simulink model "Auxiliary_Models"  (R2020b)
settings: Solver=VariableStepAuto  StartTime=0.0  StopTime=10.0  RelTol=1e-3
undefined symbols (not defined in the file or in its folder): Actuators, ampl_p_cmd, ARI, beta_cmd, Ki, Klp, Klz, Kp, Kr, omega_lp, omega_p_cmd, omega_wo, TestSequence, TrimPoint, TurnCompensation
libraries: simulink x29
settings Model: Creator=NicolasS  LastModifiedBy=NicolasS

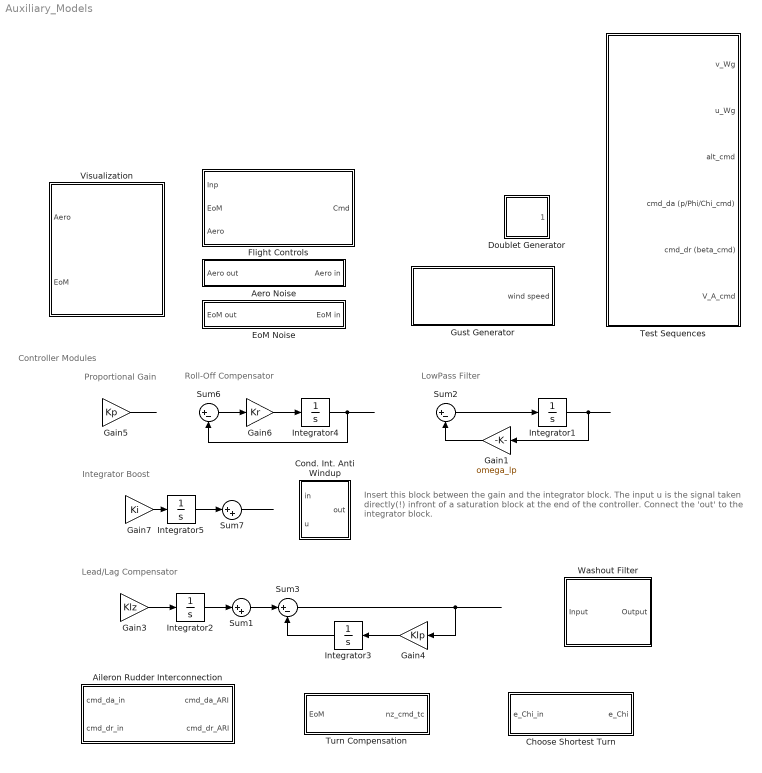
== system Auxiliary_Models ==
  note: Insert this block between the gain and the integrator block.
      | The input u is the signal taken directly(!) infront of a saturation block at the end of the controller. Connect the 'out' to the integrator block.
  note: Controller Modules
  note: Integrator Boost
  note: Roll-Off Compensator
  note: Proportional
      | Gain
  note: Lead/Lag Compensator
  note: LowPass Filter
  Aero Noise : Subsystem
  Aileron Rudder Interconnection : Subsystem
  Choose Shortest Turn : MATLAB Function  TreatAsAtomicUnit=on
  Cond. Int. Anti Windup : Subsystem  mask(Integrator Anti-Windup){max_u=inf, min_u=-inf, negative_sign=off}
      mask prompts: max_u "Maximum control signal"; min_u "Minimum control signal"; negative_sign "Negative amplification in control law"
      mask help:
      | This block provides integration using the "conditional integration" anti-windup compensation.
      | It compares the sign of the error and the sign of the control signal and stops integration in case the error drives saturation.
      mask Help:
      | This block provides integration using the "conditional integration" anti-windup compensation. It stops or continues integration depending on the sign of the integrator input (control error) and the commanded control signal. Only if the input would further increase the already saturated integrator output, integration is stopped. This method is different from "integrator clamping" and and "integrator back calculation" and usually provides better recovery properties.
      | 
      | In a standard control architecture the inputs are as follows:
      | INPUT is the error signal r-y
      | RESET is a reset signal. The integrator state is reseted on either rising or falling edges
      | X0 is the initial condition for the integrator
      | U is the commanded control signal
      | 
      | For the anti-windup to work as intended, a saturation block must be placed on the ouput of the control command being fed to the associated actuator, which should include all control signal contributions (e.g. from proportional feedback and inner loops). U is the signal before this saturation.
      | 
      | The default logic assumes a plant with positive steady-state gain to be controlled. This translates to the following logic:
      | For commanded control signal u, saturation limits Umax and Umin, and error e,
      | If u is in bounds, do nothing
      | If u >= Umax AND e > 0, stop integrating
      | If u >= Umax AND e < 0, continue integrating
      | If u <= Umin AND e > 0, continue integrating
      | If u <= Umin AND e < 0, stop integrating
      | 
      | If a plant with negative steady-state gain is to be controlled (e.g. pitch), the windup logic may changed using the NEGATIVE SIGN option. (Note: If unsure check if the controller gains are negative. If yes, check the NEGATIVE SIGN option)
      | This then translates to the logic:
      | If u is in bounds, do nothing
      | If u >= Umax AND e < 0, stop integrating
      | If u >= Umax AND e > 0, continue integrating
      | If u <= Umin AND e < 0, continue integrating
      | If u <= Umin AND e > 0, stop integrating
  Doublet Generator : Subsystem  mask(DoubletGenerator){timeon=0, pulsewidth=1, amplitude=1}
      mask prompts: timeon "Time Start"; pulsewidth "Pulse Duration"
      mask help:
      | Doublet Generator.
      | Ouputs doublet of specificed amplitude and duration.
      |
      | If start/duration/amplitude parameters are vectors, then output is multichannel.
      mask Display: plot([.1 .3 .3001 .4 .4001 .5  .5001 .7],[0 0 1 1 -1 -1 0 0])
  EoM Noise : Subsystem
  Flight Controls : Subsystem
  Gain1 : Gain  Gain=omega_lp
  Gain3 : Gain  Gain=Klz
  Gain4 : Gain  Gain=Klp
  Gain5 : Gain  Gain=Kp
  Gain6 : Gain  Gain=Kr
  Gain7 : Gain  Gain=Ki
  Gust Generator : Subsystem  mask{gust_start=0, gust_duration=0, gust_amplitude=0}
      mask prompts: gust_start "start time of the gust in sec"; gust_duration "gust duration in sec"; gust_amplitude "maximum gust speed in m/s"
      mask DialogControl ParameterGroupVar Prompt: gust characteristics
  Integrator{1..5} (5 alike) : Integrator  UpperSaturationLimit=max(Actuators.Limits.u_max_He)  LowerSaturationLimit=min(Actuators.Limits.u_max_He)  ContinuousStateAttributes='K'
  Sum1 : Sum  Inputs=|++
  Sum2 : Sum  Inputs=|+-
  Sum3 : Sum  Inputs=|+-
  Sum6 : Sum  Inputs=|+-
  Sum7 : Sum  Inputs=|++
  Test Sequences : Subsystem  InitFcn=|  StopFcn="clear beta_cmd  ampl_p_cmd omega_p_cmd tstart_p_cmd tstart_p_cmd TurnCompensation"
      | if not(exist('TestSequence','var'))
      | TestSequence = 7;
      | end
      | 
      | if not(exist('beta_cmd','var'))
      | beta_cmd = 0;
      | end
      | 
      | if not(exist('ampl_p_cmd','var'))
      | ampl_p_cmd = 0;
      | end
      | 
      | if not(exist('omega_p_cmd','var'))
      | omega_p_cmd = 0;
      | end
      | 
      | if not(exist('tstart_p_cmd','var'))
      | tstart_p_cmd = 0;
      | end
      | 
      | if not(exist('TurnCompensation','var'))
      |  if TestSequence == 4
      |     TurnCompensation = 0;
      |  else
      |     TurnCompensation = 1;
      |  end
      | end
  Turn Compensation : Subsystem
  Visualization : Subsystem
  Washout Filter : Subsystem  mask{wb=omega_wo}
      mask prompts: wb "Filter Bandwidth"
      mask Display:
      | plot([0.35 0.5 0.65 ],[0.4 0.6 0.6 ]);
      | text(0.5,0.3,[num2str(wb) ' rad/s'],'horizontalAlignment', 'center');
      | text(0.67,0.6,['1'],'horizontalAlignment', 'left');
  wires:
  Sum7/1 -> ?
  Gain7/1 -> Integrator5/1
  Sum6/1 -> Gain6/1
  Integrator5/1 -> Sum7/1
  Gain6/1 -> Integrator4/1
  ? -> Gain5/1
  ? -> Gain7/1, Sum7/2
  Gain5/1 -> ?
  ? -> Sum6/1
  Integrator4/1 -> Sum6/2
  ? -> Sum1/2, Gain3/1
  Integrator2/1 -> Sum1/1
  Sum1/1 -> Sum3/1
  Gain4/1 -> Integrator3/1
  Integrator3/1 -> Sum3/2
  Sum3/1 -> Gain4/1
  Gain3/1 -> Integrator2/1
  Gain1/1 -> Sum2/2
  Sum2/1 -> Integrator1/1
  Integrator1/1 -> Gain1/1
  ? -> Sum2/1

== system Auxiliary_Models/Aero Noise ==
  Aero in : Inport  OutDataTypeStr=Bus: Aero
  Band-Limited White Noise1 : simulink/Sources/Band-Limited White Noise  Cov=1E-7  Ts=0.01  seed=5749
  Band-Limited White Noise8 : simulink/Sources/Band-Limited White Noise  Cov=1E-7  Ts=0.01  seed=3324
  Band-Limited White Noise9 : simulink/Sources/Band-Limited White Noise  Cov=1E-3  Ts=0.05  seed=8153
  Bus Creator2 : BusCreator  Inputs=7  OutDataTypeStr=Bus: Aero
  Bus Creator3 : BusCreator  Inputs=7  OutDataTypeStr=Bus: AirData
  Bus Selector : BusSelector  OutputSignals=AirData.u_Af,AirData.v_Af,AirData.w_Af,AirData.V_A,AirData.p_dyn,AirData.alpha,AirData.beta,X_A,Y_A,Z_A,L_A,M_A,N_A
  Sum1 : Sum  Inputs=++|
  Sum2 : Sum  Inputs=++|
  Sum3 : Sum  Inputs=++|
  Aero out : Outport  OutDataTypeStr=Bus: Aero
  wires:
  Aero in/1 -> Bus Selector/1
  Bus Creator3/1 -> Bus Creator2/1  "AirData"
  Bus Selector/7 -> Sum2/2  "<beta>"
  Bus Selector/8 -> Bus Creator2/2  "<X_A>"
  Bus Creator2/1 -> Aero out/1  "Aero"
  Bus Selector/1 -> Bus Creator3/1  "<u_Af>"
  Bus Selector/3 -> Bus Creator3/3  "<w_Af>"
  Bus Selector/4 -> Sum3/2  "<V_A>"
  Bus Selector/6 -> Sum1/2  "<alpha>"
  Band-Limited White Noise8/1 -> Sum1/1
  Sum1/1 -> Bus Creator3/6  "alpha"
  Bus Selector/5 -> Bus Creator3/5  "<p_dyn>"
  Band-Limited White Noise9/1 -> Sum3/1
  Sum3/1 -> Bus Creator3/4  "V_A"
  Bus Selector/2 -> Bus Creator3/2  "<v_Af>"
  Bus Selector/9 -> Bus Creator2/3  "<Y_A>"
  Bus Selector/10 -> Bus Creator2/4  "<Z_A>"
  Bus Selector/11 -> Bus Creator2/5  "<L_A>"
  Bus Selector/12 -> Bus Creator2/6  "<M_A>"
  Bus Selector/13 -> Bus Creator2/7  "<N_A>"
  Band-Limited White Noise1/1 -> Sum2/1
  Sum2/1 -> Bus Creator3/7  "beta"

== system Auxiliary_Models/Aileron Rudder Interconnection ==
  cmd_da_in : Inport
  cmd_dr_in : Inport  Port=2
  ARI : Constant  Value=ARI
  Demux : Demux  Outputs=2
  Mux : Mux  Inputs=2
  Product : Product  Multiplication=Matrix(*)
  cmd_da_ARI : Outport
  cmd_dr_ARI : Outport  Port=2
  wires:
  cmd_da_in/1 -> Mux/1
  ARI/1 -> Product/1
  Demux/1 -> cmd_da_ARI/1
  Demux/2 -> cmd_dr_ARI/1
  Product/1 -> Demux/1
  cmd_dr_in/1 -> Mux/2
  Mux/1 -> Product/2

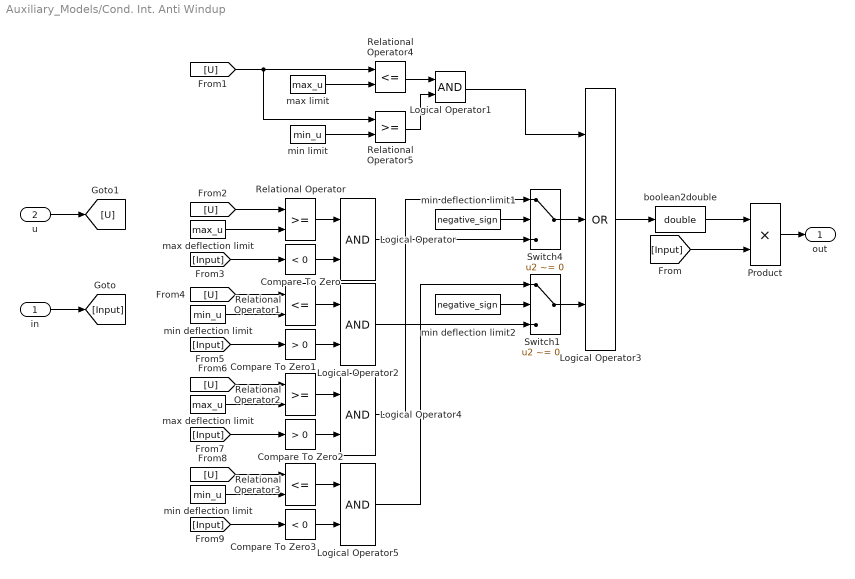
== system Auxiliary_Models/Cond. Int. Anti Windup ==
  in : Inport
  u : Inport  Port=2
  Compare To Zero : simulink/Logic and Bit Operations/Compare To Zero  relop=<  OutDataTypeStr=uint8
  Compare To Zero1 : simulink/Logic and Bit Operations/Compare To Zero  relop=>  OutDataTypeStr=uint8
  Compare To Zero2 : simulink/Logic and Bit Operations/Compare To Zero  relop=>  OutDataTypeStr=uint8
  Compare To Zero3 : simulink/Logic and Bit Operations/Compare To Zero  relop=<  OutDataTypeStr=uint8
  Logical Operator{,1..2,4..5} (5 alike) : Logic  AllPortsSameDT=off  OutDataTypeStr=boolean
  Logical Operator3 : Logic  Operator=OR  Inputs=3  AllPortsSameDT=off  OutDataTypeStr=boolean
  Product : Product
  Relational Operator : RelationalOperator  OutDataTypeStr=boolean  RndMeth=Nearest
  Relational Operator1 : RelationalOperator  Operator=<=  OutDataTypeStr=boolean  RndMeth=Nearest
  Relational Operator2 : RelationalOperator  OutDataTypeStr=boolean  RndMeth=Nearest
  Relational Operator3 : RelationalOperator  Operator=<=  OutDataTypeStr=boolean  RndMeth=Nearest
  Relational Operator4 : RelationalOperator  Operator=<=  OutDataTypeStr=boolean  RndMeth=Nearest
  Relational Operator5 : RelationalOperator  OutDataTypeStr=boolean  RndMeth=Nearest
  Switch1 : Switch  Criteria=u2 ~= 0
  Switch4 : Switch  Criteria=u2 ~= 0
  boolean2double : DataTypeConversion  OutDataTypeStr=double
  max deflection limit : Constant  Value=max_u  SampleTime=-1
  "max deflection limit " : Constant  Value=max_u  SampleTime=-1
  max limit : Constant  Value=max_u  SampleTime=-1
  min deflection limit : Constant  Value=min_u  SampleTime=-1
  "min deflection limit " : Constant  Value=min_u  SampleTime=-1
  min deflection limit1 : Constant  Value=negative_sign  SampleTime=-1
  min deflection limit2 : Constant  Value=negative_sign  SampleTime=-1
  min limit : Constant  Value=min_u  SampleTime=-1
  out : Outport
  wires:
  Product/1 -> out/1
  Logical Operator3/1 -> boolean2double/1
  boolean2double/1 -> Product/1
  [Input] -> Product/2
  [Input] -> Compare To Zero3/1
  [U] -> Relational Operator3/1
  [Input] -> Compare To Zero2/1
  [U] -> Relational Operator2/1
  [Input] -> Compare To Zero1/1
  [U] -> Relational Operator1/1
  [Input] -> Compare To Zero/1
  [U] -> Relational Operator/1
  [U] -> Relational Operator4/1, Relational Operator5/1
  u/1 -> [U]
  in/1 -> [Input]
  min limit/1 -> Relational Operator5/2
  Relational Operator5/1 -> Logical Operator1/2
  Relational Operator4/1 -> Logical Operator1/1
  max limit/1 -> Relational Operator4/2
  Logical Operator5/1 -> Switch1/1
  Logical Operator4/1 -> Switch4/1
  Logical Operator2/1 -> Switch1/3
  Logical Operator/1 -> Switch4/3
  min deflection limit1/1 -> Switch4/2
  Switch1/1 -> Logical Operator3/3
  min deflection limit2/1 -> Switch1/2
  max deflection limit/1 -> Relational Operator/2
  Compare To Zero/1 -> Logical Operator/2
  Relational Operator/1 -> Logical Operator/1
  Compare To Zero1/1 -> Logical Operator2/2
  Relational Operator1/1 -> Logical Operator2/1
  min deflection limit/1 -> Relational Operator1/2
  Switch4/1 -> Logical Operator3/2
  Logical Operator1/1 -> Logical Operator3/1
  Compare To Zero2/1 -> Logical Operator4/2
  Relational Operator2/1 -> Logical Operator4/1
  Compare To Zero3/1 -> Logical Operator5/2
  Relational Operator3/1 -> Logical Operator5/1
  "min deflection limit "/1 -> Relational Operator3/2
  "max deflection limit "/1 -> Relational Operator2/2

== system Auxiliary_Models/Doublet Generator ==
  Add : Sum  Inputs=+++
  DownStep : Step  Time=timeon+pulsewidth  After=-2  SampleTime=0
  Gain : Gain  Gain=amplitude
  UnStep : Step  Time=timeon+2*pulsewidth  SampleTime=0
  UpStep : Step  Time=timeon  SampleTime=0
  Doublet : Outport
  wires:
  UpStep/1 -> Add/1
  DownStep/1 -> Add/2
  UnStep/1 -> Add/3
  Add/1 -> Gain/1
  Gain/1 -> Doublet/1

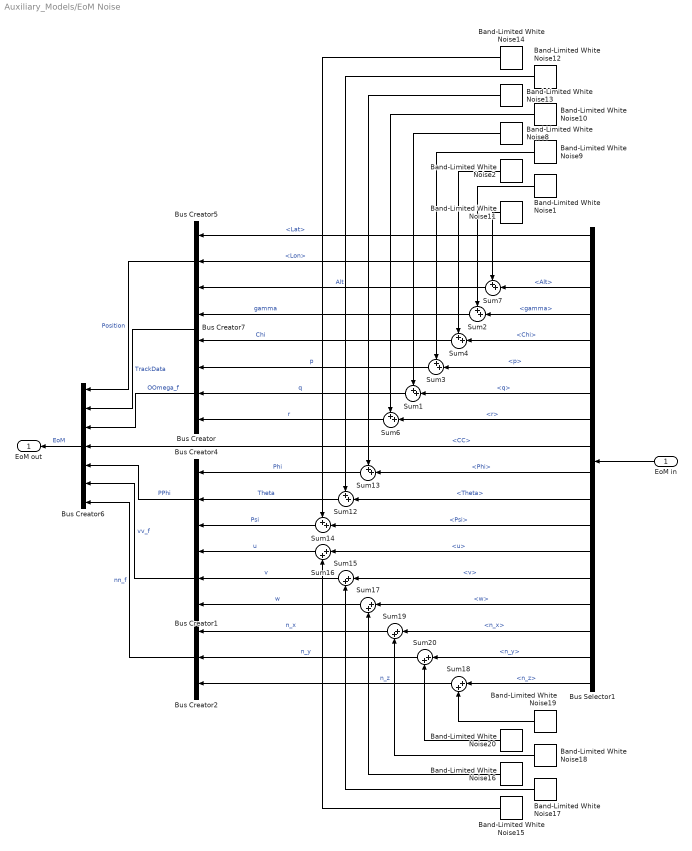
== system Auxiliary_Models/EoM Noise ==
  EoM in : Inport  OutDataTypeStr=Bus: EoM
  Band-Limited White Noise1 : simulink/Sources/Band-Limited White Noise  Cov=1E-7  Ts=0.01  seed=1102
  Band-Limited White Noise10 : simulink/Sources/Band-Limited White Noise  Cov=1E-6  Ts=0.01  seed=66897
  Band-Limited White Noise11 : simulink/Sources/Band-Limited White Noise  Cov=1E-4  Ts=0.1  seed=6874
  Band-Limited White Noise12 : simulink/Sources/Band-Limited White Noise  Cov=5E-7  Ts=0.01  seed=45875
  Band-Limited White Noise13 : simulink/Sources/Band-Limited White Noise  Cov=5E-7  Ts=0.01  seed=74148
  Band-Limited White Noise14 : simulink/Sources/Band-Limited White Noise  Cov=5E-7  Ts=0.01  seed=3514
  Band-Limited White Noise15 : simulink/Sources/Band-Limited White Noise  Cov=5E-5  Ts=0.1  seed=54769
  Band-Limited White Noise16 : simulink/Sources/Band-Limited White Noise  Cov=1E-4  Ts=0.01  seed=6932
  Band-Limited White Noise17 : simulink/Sources/Band-Limited White Noise  Cov=1E-4  Ts=0.01  seed=4485
  Band-Limited White Noise18 : simulink/Sources/Band-Limited White Noise  Cov=1E-5  Ts=0.01  seed=11452
  Band-Limited White Noise19 : simulink/Sources/Band-Limited White Noise  Cov=1E-5  Ts=0.01  seed=3324
  Band-Limited White Noise2 : simulink/Sources/Band-Limited White Noise  Cov=1E-7  Ts=0.1  seed=2201
  Band-Limited White Noise20 : simulink/Sources/Band-Limited White Noise  Cov=1E-5  Ts=0.01  seed=58967
  Band-Limited White Noise8 : simulink/Sources/Band-Limited White Noise  Cov=1E-6  Ts=0.01  seed=[23341]
  Band-Limited White Noise9 : simulink/Sources/Band-Limited White Noise  Cov=1E-6  Ts=0.01  seed=1147
  Bus Creator : BusCreator  Inputs=3  OutDataTypeStr=Bus: OOmega_f
  Bus Creator1 : BusCreator  Inputs=3  OutDataTypeStr=Bus: vv_f
  Bus Creator2 : BusCreator  Inputs=3  OutDataTypeStr=Bus: nn_f
  Bus Creator4 : BusCreator  Inputs=3  OutDataTypeStr=Bus: PPhi
  Bus Creator5 : BusCreator  Inputs=3  OutDataTypeStr=Bus: Position
  Bus Creator6 : BusCreator  Inputs=7  OutDataTypeStr=Bus: EoM
  Bus Creator7 : BusCreator  Inputs=2  OutDataTypeStr=Bus: TrackData
  Bus Selector1 : BusSelector  OutputSignals=Position.Lat,Position.Lon,Position.Alt,TrackData.gamma,TrackData.Chi,OOmega_f.p,OOmega_f.q,OOmega_f.r,CC,PPhi.Phi,PPhi.Theta,PPhi.Psi,vv_f.u,vv_f.v,vv_f.w,nn_f.n_x,nn_f.n_y,nn_f.n_z
  Sum{1..4,6..7,12..14} (9 alike) : Sum  Inputs=++|
  Sum{15..20} (6 alike) : Sum  Inputs=|++
  EoM out : Outport  OutDataTypeStr=Bus: EoM
  wires:
  EoM in/1 -> Bus Selector1/1
  Bus Selector1/6 -> Sum3/2  "<p>"
  Bus Selector1/7 -> Sum1/2  "<q>"
  Band-Limited White Noise9/1 -> Sum3/1
  Bus Selector1/8 -> Sum6/2  "<r>"
  Band-Limited White Noise10/1 -> Sum6/1
  Band-Limited White Noise11/1 -> Sum7/1
  Bus Selector1/3 -> Sum7/2  "<Alt>"
  Band-Limited White Noise12/1 -> Sum12/1
  Bus Selector1/10 -> Sum13/2  "<Phi>"
  Bus Selector1/11 -> Sum12/2  "<Theta>"
  Bus Selector1/12 -> Sum14/2  "<Psi>"
  Band-Limited White Noise13/1 -> Sum13/1
  Band-Limited White Noise14/1 -> Sum14/1
  Bus Selector1/16 -> Sum19/1  "<n_x>"
  Bus Selector1/17 -> Sum20/1  "<n_y>"
  Bus Selector1/18 -> Sum18/1  "<n_z>"
  Bus Selector1/15 -> Sum17/1  "<w>"
  Bus Selector1/13 -> Sum16/1  "<u>"
  Band-Limited White Noise16/1 -> Sum17/2
  Band-Limited White Noise15/1 -> Sum16/2
  Bus Selector1/14 -> Sum15/1  "<v>"
  Band-Limited White Noise17/1 -> Sum15/2
  Band-Limited White Noise19/1 -> Sum18/2
  Band-Limited White Noise18/1 -> Sum19/2
  Band-Limited White Noise20/1 -> Sum20/2
  Bus Selector1/1 -> Bus Creator5/1  "<Lat>"
  Bus Selector1/2 -> Bus Creator5/2  "<Lon>"
  Sum19/1 -> Bus Creator2/1  "n_x"
  Sum20/1 -> Bus Creator2/2  "n_y"
  Sum18/1 -> Bus Creator2/3  "n_z"
  Sum15/1 -> Bus Creator1/2  "v"
  Sum16/1 -> Bus Creator1/1  "u"
  Sum17/1 -> Bus Creator1/3  "w"
  Sum7/1 -> Bus Creator5/3  "Alt"
  Sum6/1 -> Bus Creator/3  "r"
  Sum1/1 -> Bus Creator/2  "q"
  Sum3/1 -> Bus Creator/1  "p"
  Sum13/1 -> Bus Creator4/1  "Phi"
  Bus Selector1/9 -> Bus Creator6/4  "<CC>"
  Sum12/1 -> Bus Creator4/2  "Theta"
  Sum14/1 -> Bus Creator4/3  "Psi"
  Bus Creator5/1 -> Bus Creator6/1  "Position"
  Bus Creator/1 -> Bus Creator6/3  "OOmega_f"
  Bus Creator4/1 -> Bus Creator6/5  "PPhi"
  Bus Creator1/1 -> Bus Creator6/6  "vv_f"
  Bus Creator2/1 -> Bus Creator6/7  "nn_f"
  Bus Creator6/1 -> EoM out/1  "EoM"
  Band-Limited White Noise8/1 -> Sum1/1
  Bus Creator7/1 -> Bus Creator6/2  "TrackData"
  Band-Limited White Noise1/1 -> Sum2/1
  Bus Selector1/5 -> Sum4/2  "<Chi>"
  Band-Limited White Noise2/1 -> Sum4/1
  Bus Selector1/4 -> Sum2/2  "<gamma>"
  Sum2/1 -> Bus Creator7/1  "gamma"
  Sum4/1 -> Bus Creator7/2  "Chi"

== system Auxiliary_Models/Flight Controls ==
  Inp : Inport
  EoM : Inport  Port=2  OutDataTypeStr=Bus: EoM
  Aero : Inport  Port=3  OutDataTypeStr=Bus: Aero
  Bus Creator1 : BusCreator  Inputs=4  OutDataTypeStr=Bus: Cmd
  Lateral Directional Control Laws : Subsystem
  Longitudinal Control Laws : Subsystem
  Cmd : Outport  OutDataTypeStr=Bus: Cmd
  wires:
  Inp/1 -> Lateral Directional Control Laws/3(Inp), Longitudinal Control Laws/3(Inp)
  Bus Creator1/1 -> Cmd/1  "Cmd"
  Lateral Directional Control Laws/2(cmd_dr) -> Bus Creator1/3  "cmd_dr"
  EoM/1 -> Lateral Directional Control Laws/2(EoM), Longitudinal Control Laws/2(EoM)
  Longitudinal Control Laws/1(cmd_de) -> Bus Creator1/1  "cmd_de"
  Lateral Directional Control Laws/1(cmd_da) -> Bus Creator1/2  "cmd_da"
  Longitudinal Control Laws/2(cmd_dt) -> Bus Creator1/4  "cmd_dt"
  Aero/1 -> Lateral Directional Control Laws/1(Aero), Longitudinal Control Laws/1(Aero)

== system Auxiliary_Models/Gust Generator ==
  1-cos gust : Subsystem  TreatAsAtomicUnit=on
  Clock : Clock
  Compare To Constant : simulink/Logic and Bit Operations/Compare To Constant  relop=>=  const=gust_start  OutDataTypeStr=boolean
  Constant : Constant  Value=0
  Sum : Sum  Inputs=+-|
  Switch : Switch  Criteria=u2 > Threshold  Threshold=gust_start+gust_duration
  time freeze : Subsystem  TreatAsAtomicUnit=on
  wind speed : Outport
  wires:
  time freeze/1(out) -> Sum/2
  Constant/1 -> Switch/1
  Clock/1 -> time freeze/1(in), Compare To Constant/1, Sum/1, Switch/2
  Compare To Constant/1 -> 1-cos gust/Enable, time freeze/Trigger
  Sum/1 -> 1-cos gust/1(in)
  1-cos gust/1(wind) -> Switch/3
  Switch/1 -> wind speed/1

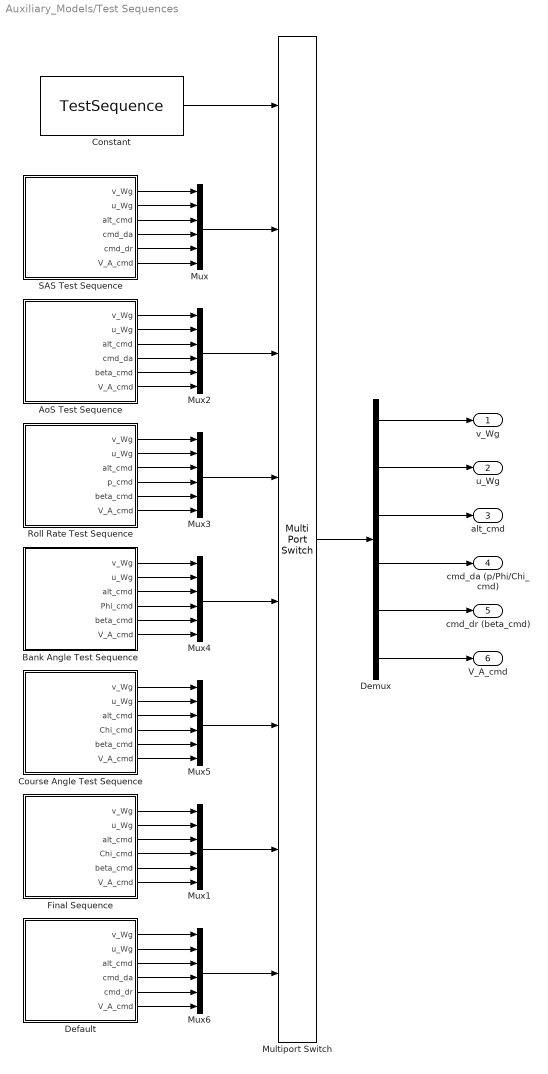
== system Auxiliary_Models/Test Sequences ==
  AoS Test Sequence : Subsystem
  Bank Angle Test Sequence : Subsystem
  Constant : Constant  Value=TestSequence
  Course Angle Test Sequence : Subsystem
  Default : Subsystem
  Demux : Demux  Outputs=6
  Final Sequence : Subsystem
  Multiport Switch : MultiPortSwitch  Inputs=7
  Mux{,1..6} (7 alike) : Mux  Inputs=6
  Roll Rate Test Sequence : Subsystem
  SAS Test Sequence : Subsystem
  v_Wg : Outport
  u_Wg : Outport  Port=2
  alt_cmd : Outport  Port=3
  cmd_da (p/Phi/Chi_cmd) : Outport  Port=4
  cmd_dr (beta_cmd) : Outport  Port=5
  V_A_cmd : Outport  Port=6
  wires:
  SAS Test Sequence/1(v_Wg) -> Mux/1
  SAS Test Sequence/2(u_Wg) -> Mux/2
  SAS Test Sequence/3(alt_cmd) -> Mux/3
  SAS Test Sequence/4(cmd_da) -> Mux/4
  SAS Test Sequence/5(cmd_dr) -> Mux/5
  SAS Test Sequence/6(V_A_cmd) -> Mux/6
  Final Sequence/1(v_Wg) -> Mux1/1
  Final Sequence/2(u_Wg) -> Mux1/2
  Final Sequence/3(alt_cmd) -> Mux1/3
  Final Sequence/4(Chi_cmd) -> Mux1/4
  Final Sequence/5(beta_cmd) -> Mux1/5
  Final Sequence/6(V_A_cmd) -> Mux1/6
  AoS Test Sequence/6(V_A_cmd) -> Mux2/6
  AoS Test Sequence/5(beta_cmd) -> Mux2/5
  AoS Test Sequence/4(cmd_da) -> Mux2/4
  AoS Test Sequence/3(alt_cmd) -> Mux2/3
  AoS Test Sequence/2(u_Wg) -> Mux2/2
  AoS Test Sequence/1(v_Wg) -> Mux2/1
  Roll Rate Test Sequence/1(v_Wg) -> Mux3/1
  Roll Rate Test Sequence/5(beta_cmd) -> Mux3/5
  Roll Rate Test Sequence/2(u_Wg) -> Mux3/2
  Roll Rate Test Sequence/4(p_cmd) -> Mux3/4
  Roll Rate Test Sequence/3(alt_cmd) -> Mux3/3
  Roll Rate Test Sequence/6(V_A_cmd) -> Mux3/6
  Bank Angle Test Sequence/1(v_Wg) -> Mux4/1
  Bank Angle Test Sequence/2(u_Wg) -> Mux4/2
  Bank Angle Test Sequence/3(alt_cmd) -> Mux4/3
  Bank Angle Test Sequence/4(Phi_cmd) -> Mux4/4
  Bank Angle Test Sequence/5(beta_cmd) -> Mux4/5
  Bank Angle Test Sequence/6(V_A_cmd) -> Mux4/6
  Course Angle Test Sequence/4(Chi_cmd) -> Mux5/4
  Course Angle Test Sequence/5(beta_cmd) -> Mux5/5
  Course Angle Test Sequence/2(u_Wg) -> Mux5/2
  Course Angle Test Sequence/1(v_Wg) -> Mux5/1
  Course Angle Test Sequence/3(alt_cmd) -> Mux5/3
  Course Angle Test Sequence/6(V_A_cmd) -> Mux5/6
  Multiport Switch/1 -> Demux/1
  Demux/1 -> v_Wg/1
  Demux/2 -> u_Wg/1
  Demux/3 -> alt_cmd/1
  Demux/4 -> cmd_da (p/Phi/Chi_cmd)/1
  Demux/5 -> cmd_dr (beta_cmd)/1
  Demux/6 -> V_A_cmd/1
  Mux/1 -> Multiport Switch/2
  Mux2/1 -> Multiport Switch/3
  Mux3/1 -> Multiport Switch/4
  Mux4/1 -> Multiport Switch/5
  Mux5/1 -> Multiport Switch/6
  Constant/1 -> Multiport Switch/1
  Default/6(V_A_cmd) -> Mux6/6
  Default/5(cmd_dr) -> Mux6/5
  Default/4(cmd_da) -> Mux6/4
  Default/3(alt_cmd) -> Mux6/3
  Default/2(u_Wg) -> Mux6/2
  Default/1(v_Wg) -> Mux6/1
  Mux1/1 -> Multiport Switch/7
  Mux6/1 -> Multiport Switch/8

== system Auxiliary_Models/Turn Compensation ==
  note: this gain block is parameterized via the matlab live script and used to switch the turn compensation on or off
  EoM : Inport  OutDataTypeStr=Bus: EoM
  Gain : Gain  Gain=TurnCompensation
  nz_cmd_tc : Outport
  wires:
  Gain/1 -> nz_cmd_tc/1  "nz_cmd_tc"

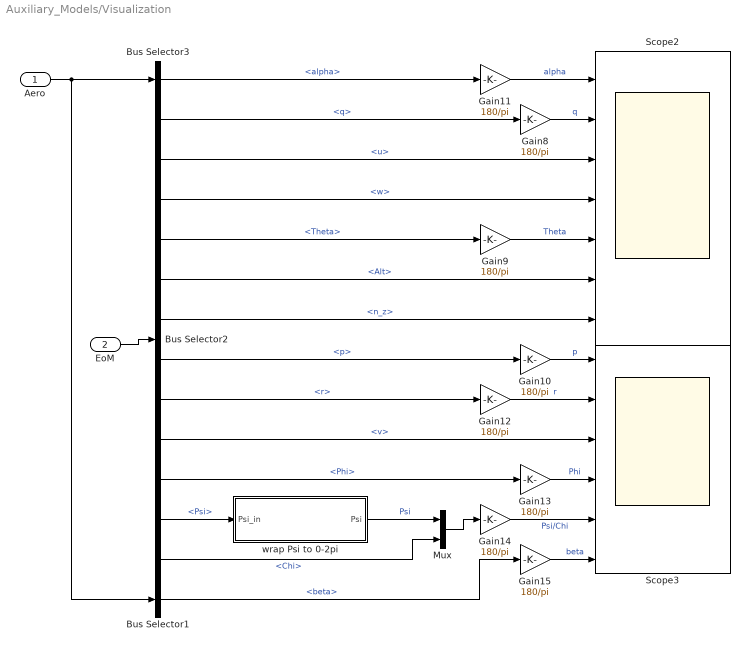
== system Auxiliary_Models/Visualization ==
  Aero : Inport  OutDataTypeStr=Bus: Aero
  EoM : Inport  Port=2  OutDataTypeStr=Bus: EoM
  Bus Selector1 : BusSelector  OutputSignals=AirData.beta
  Bus Selector2 : BusSelector  OutputSignals=OOmega_f.q,vv_f.u,vv_f.w,PPhi.Theta,Position.Alt,nn_f.n_z,OOmega_f.p,OOmega_f.r,vv_f.v,PPhi.Phi,PPhi.Psi,TrackData.Chi
  Bus Selector3 : BusSelector  OutputSignals=AirData.alpha
  Gain{8..15} (8 alike) : Gain  Gain=180/pi
  Mux : Mux  Inputs=2
  Scope2 : Scope  NumInputPorts=7
  Scope3 : Scope  NumInputPorts=6
  wrap Psi to 0-2pi : MATLAB Function  TreatAsAtomicUnit=on
  wires:
  Bus Selector2/8 -> Gain12/1  "<r>"
  Gain8/1 -> Scope2/2  "q"
  Gain13/1 -> Scope3/4  "Phi"
  Gain12/1 -> Scope3/2  "r"
  Gain15/1 -> Scope3/6  "beta"
  Gain11/1 -> Scope2/1  "alpha"
  Gain14/1 -> Scope3/5  "Psi/Chi"
  Gain9/1 -> Scope2/5  "Theta"
  Gain10/1 -> Scope3/1  "p"
  Aero/1 -> Bus Selector3/1, Bus Selector1/1
  Bus Selector2/9 -> Scope3/3  "<v>"
  Bus Selector2/2 -> Scope2/3  "<u>"
  Bus Selector2/1 -> Gain8/1  "<q>"
  EoM/1 -> Bus Selector2/1
  Bus Selector2/6 -> Scope2/7  "<n_z>"
  Bus Selector2/11 -> wrap Psi to 0-2pi/1(Psi_in)  "<Psi>"
  Bus Selector2/5 -> Scope2/6  "<Alt>"
  Bus Selector3/1 -> Gain11/1  "<alpha>"
  Bus Selector2/10 -> Gain13/1  "<Phi>"
  Bus Selector2/3 -> Scope2/4  "<w>"
  Bus Selector2/7 -> Gain10/1  "<p>"
  Bus Selector2/4 -> Gain9/1  "<Theta>"
  Bus Selector1/1 -> Gain15/1  "<beta>"
  Bus Selector2/12 -> Mux/2  "<Chi>"
  Mux/1 -> Gain14/1
  wrap Psi to 0-2pi/1(Psi) -> Mux/1  "Psi"

== system Auxiliary_Models/Washout Filter ==
  Input : Inport
  Gain : Gain  Gain=wb
  Gain1 : Gain  Gain=wb
  Integrator : Integrator  ContinuousStateAttributes='K_wo'
  Sum3 : Sum  Inputs=++|
  Sum5 : Sum  Inputs=|--
  Output : Outport
  wires:
  Gain/1 -> Sum5/2
  Integrator/1 -> Gain/1, Sum3/2
  Input/1 -> Gain1/1, Sum3/1
  Sum5/1 -> Integrator/1
  Gain1/1 -> Sum5/1
  Sum3/1 -> Output/1

== system Auxiliary_Models/Flight Controls/Lateral Directional Control Laws ==
  Aero : Inport  OutDataTypeStr=Bus: Aero
  EoM : Inport  Port=2  OutDataTypeStr=Bus: EoM
  Inp : Inport  Port=3
  Demux : Demux  Outputs=2
  Saturation : Saturate  UpperLimit=max(Actuators.Limits.u_max_Hr)  LowerLimit=min(Actuators.Limits.u_max_Hr)
  Saturation1 : Saturate  UpperLimit=max(Actuators.Limits.u_max_Ha)  LowerLimit=min(Actuators.Limits.u_max_Ha)
  Selector : Selector  InputPortWidth=4  IndexOptions=Index vector (dialog)  Indices=[2 3]  OutputSizes=1
  Terminator1 : Terminator
  Terminator3 : Terminator
  cmd_da : Outport
  cmd_dr : Outport  Port=2
  wires:
  EoM/1 -> Terminator3/1
  Inp/1 -> Selector/1  "Inp"
  Aero/1 -> Terminator1/1
  Demux/1 -> Saturation1/1
  Selector/1 -> Demux/1
  Saturation1/1 -> cmd_da/1  "cmd_da"
  Demux/2 -> Saturation/1
  Saturation/1 -> cmd_dr/1  "cmd_dr"

== system Auxiliary_Models/Flight Controls/Longitudinal Control Laws ==
  Aero : Inport  OutDataTypeStr=Bus: Aero
  EoM : Inport  Port=2  OutDataTypeStr=Bus: EoM
  Inp : Inport  Port=3
  Demux : Demux  Outputs=2
  Saturation : Saturate  UpperLimit=1  LowerLimit=0
  Saturation1 : Saturate  UpperLimit=max(Actuators.Limits.u_max_He)  LowerLimit=min(Actuators.Limits.u_max_He)
  Selector : Selector  InputPortWidth=4  IndexOptions=Index vector (dialog)  Indices=[1 4]  OutputSizes=1
  Terminator : Terminator
  Terminator2 : Terminator
  cmd_de : Outport
  cmd_dt : Outport  Port=2
  wires:
  Inp/1 -> Selector/1  "Inp"
  Selector/1 -> Demux/1
  EoM/1 -> Terminator/1
  Aero/1 -> Terminator2/1
  Demux/2 -> Saturation/1
  Demux/1 -> Saturation1/1
  Saturation1/1 -> cmd_de/1  "cmd_de"
  Saturation/1 -> cmd_dt/1  "cmd_dt"

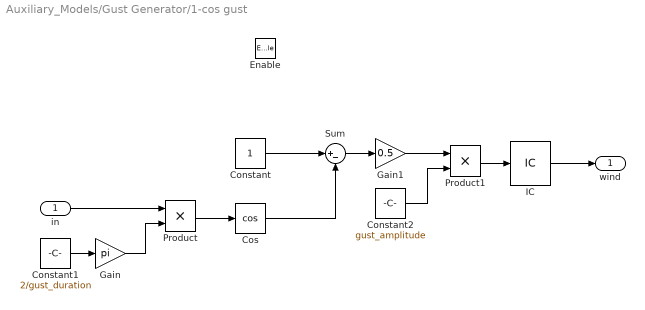
== system Auxiliary_Models/Gust Generator/1-cos gust ==
  in : Inport
  Enable : EnablePort  StatesWhenEnabling=reset
  Constant : Constant
  Constant1 : Constant  Value=2/gust_duration
  Constant2 : Constant  Value=gust_amplitude
  Cos : Trigonometry  Operator=cos
  Gain : Gain  Gain=pi
  Gain1 : Gain  Gain=0.5
  IC : InitialCondition  Value=0
  Product : Product
  Product1 : Product
  Sum : Sum  Inputs=|+-
  wind : Outport
  wires:
  IC/1 -> wind/1
  Constant1/1 -> Gain/1
  Product1/1 -> IC/1
  Product/1 -> Cos/1
  Cos/1 -> Sum/2
  Constant/1 -> Sum/1
  Gain/1 -> Product/2
  Gain1/1 -> Product1/1
  Sum/1 -> Gain1/1
  Constant2/1 -> Product1/2
  in/1 -> Product/1

== system Auxiliary_Models/Gust Generator/time freeze ==
  in : Inport
  Trigger : TriggerPort  VariantControl=Variant
  out : Outport  InitialOutput=0
  wires:
  in/1 -> out/1

== system Auxiliary_Models/Test Sequences/AoS Test Sequence ==
  Constant : Constant  Value=TrimPoint.States.Altbar
  Constant1 : Constant  Value=sqrt(TrimPoint.States.ubar^2+TrimPoint.States.vbar^2+TrimPoint.States.wbar^2)
  Constant2 : Constant  Value=TrimPoint.States.dabar
  Constant3 : Constant  Value=0
  Gust Generator : Subsystem  mask{gust_start=5, gust_duration=25, gust_amplitude=-30}
      mask prompts: gust_start "start time of the gust in sec"; gust_duration "gust duration in sec"; gust_amplitude "maximum gust speed in m/s"
      mask DialogControl ParameterGroupVar Prompt: gust characteristics
  Step : Step  Time=40  After=beta_cmd  SampleTime=0
  v_Wg : Outport
  u_Wg : Outport  Port=2
  alt_cmd : Outport  Port=3
  cmd_da : Outport  Port=4
  beta_cmd : Outport  Port=5
  V_A_cmd : Outport  Port=6
  wires:
  Constant3/1 -> u_Wg/1  "u_Wg"
  Constant2/1 -> cmd_da/1  "cmd_da"
  Constant1/1 -> V_A_cmd/1  "V_A_cmd"
  Step/1 -> beta_cmd/1  "beta_cmd"
  Constant/1 -> alt_cmd/1  "alt_cmd"
  Gust Generator/1(wind speed) -> v_Wg/1  "v_Wg"

== system Auxiliary_Models/Test Sequences/Bank Angle Test Sequence ==
  Constant : Constant  Value=TrimPoint.States.Altbar
  Constant1 : Constant  Value=sqrt(TrimPoint.States.ubar^2+TrimPoint.States.vbar^2+TrimPoint.States.wbar^2)
  Constant2 : Constant  Value=0
  Constant3 : Constant  Value=0
  Doublet Generator : Subsystem  mask(DoubletGenerator){timeon=5, pulsewidth=20, amplitude=deg2rad(55)}
      mask prompts: timeon "Time Start"; pulsewidth "Pulse Duration"
      mask help:
      | Doublet Generator.
      | Ouputs doublet of specificed amplitude and duration.
      |
      | If start/duration/amplitude parameters are vectors, then output is multichannel.
      mask Display: plot([.1 .3 .3001 .4 .4001 .5  .5001 .7],[0 0 1 1 -1 -1 0 0])
  Gust Generator : Subsystem  mask{gust_start=5, gust_duration=25, gust_amplitude=-30}
      mask prompts: gust_start "start time of the gust in sec"; gust_duration "gust duration in sec"; gust_amplitude "maximum gust speed in m/s"
      mask DialogControl ParameterGroupVar Prompt: gust characteristics
  v_Wg : Outport
  u_Wg : Outport  Port=2
  alt_cmd : Outport  Port=3
  Phi_cmd : Outport  Port=4
  beta_cmd : Outport  Port=5
  V_A_cmd : Outport  Port=6
  wires:
  Constant3/1 -> u_Wg/1  "u_Wg"
  Doublet Generator/1(Doublet) -> Phi_cmd/1  "Phi_cmd"
  Constant1/1 -> V_A_cmd/1  "V_A_cmd"
  Constant2/1 -> beta_cmd/1  "beta_cmd"
  Constant/1 -> alt_cmd/1  "alt_cmd"
  Gust Generator/1(wind speed) -> v_Wg/1  "v_Wg"

== system Auxiliary_Models/Test Sequences/Course Angle Test Sequence ==
  Constant : Constant  Value=TrimPoint.States.Altbar
  Constant1 : Constant  Value=sqrt(TrimPoint.States.ubar^2+TrimPoint.States.vbar^2+TrimPoint.States.wbar^2)
  Constant2 : Constant  Value=0
  Constant3 : Constant  Value=0
  Gust Generator : Subsystem  mask{gust_start=40, gust_duration=25, gust_amplitude=-30}
      mask prompts: gust_start "start time of the gust in sec"; gust_duration "gust duration in sec"; gust_amplitude "maximum gust speed in m/s"
      mask DialogControl ParameterGroupVar Prompt: gust characteristics
  Step1 : Step  Time=10  Before=TrimPoint.States.Psibar  After=deg2rad(350)  SampleTime=0
  v_Wg : Outport
  u_Wg : Outport  Port=2
  alt_cmd : Outport  Port=3
  Chi_cmd : Outport  Port=4
  beta_cmd : Outport  Port=5
  V_A_cmd : Outport  Port=6
  wires:
  Constant3/1 -> u_Wg/1  "u_Wg"
  Step1/1 -> Chi_cmd/1  "Chi_cmd"
  Constant1/1 -> V_A_cmd/1  "V_A_cmd"
  Constant2/1 -> beta_cmd/1  "beta_cmd"
  Constant/1 -> alt_cmd/1  "alt_cmd"
  Gust Generator/1(wind speed) -> v_Wg/1  "v_Wg"

== system Auxiliary_Models/Test Sequences/Default ==
  Constant : Constant  Value=TrimPoint.States.Altbar
  Constant1 : Constant  Value=sqrt(TrimPoint.States.ubar^2+TrimPoint.States.vbar^2+TrimPoint.States.wbar^2)
  Constant2 : Constant  Value=TrimPoint.States.dabar
  Constant3 : Constant  Value=0
  Constant4 : Constant  Value=TrimPoint.States.drbar
  Constant5 : Constant  Value=0
  v_Wg : Outport
  u_Wg : Outport  Port=2
  alt_cmd : Outport  Port=3
  cmd_da : Outport  Port=4
  cmd_dr : Outport  Port=5
  V_A_cmd : Outport  Port=6
  wires:
  Constant/1 -> alt_cmd/1  "alt_cmd"
  Constant1/1 -> V_A_cmd/1  "V_A_cmd"
  Constant2/1 -> cmd_da/1  "cmd_da"
  Constant4/1 -> cmd_dr/1  "cmd_dr"
  Constant5/1 -> v_Wg/1  "v_Wg"
  Constant3/1 -> u_Wg/1  "u_Wg"

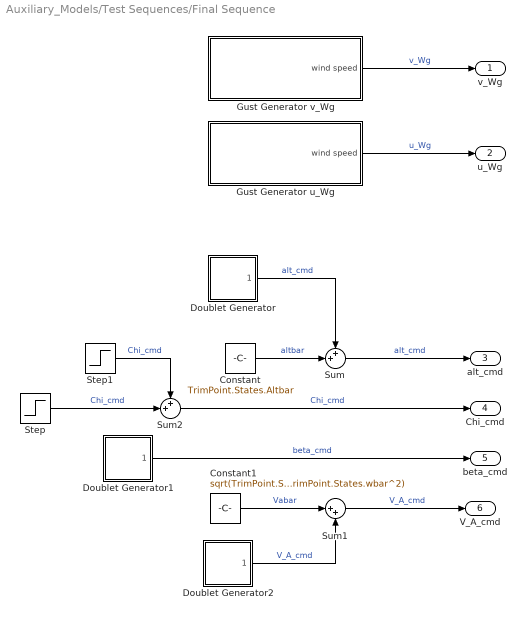
== system Auxiliary_Models/Test Sequences/Final Sequence ==
  Constant : Constant  Value=TrimPoint.States.Altbar
  Constant1 : Constant  Value=sqrt(TrimPoint.States.ubar^2+TrimPoint.States.vbar^2+TrimPoint.States.wbar^2)
  Doublet Generator : Subsystem  mask(DoubletGenerator){timeon=15, pulsewidth=40, amplitude=200}
      mask prompts: timeon "Time Start"; pulsewidth "Pulse Duration"
      mask help:
      | Doublet Generator.
      | Ouputs doublet of specificed amplitude and duration.
      |
      | If start/duration/amplitude parameters are vectors, then output is multichannel.
      mask Display: plot([.1 .3 .3001 .4 .4001 .5  .5001 .7],[0 0 1 1 -1 -1 0 0])
  Doublet Generator1 : Subsystem  mask(DoubletGenerator){timeon=60, pulsewidth=20, amplitude=deg2rad(3)}
      mask prompts: timeon "Time Start"; pulsewidth "Pulse Duration"
      mask help:
      | Doublet Generator.
      | Ouputs doublet of specificed amplitude and duration.
      |
      | If start/duration/amplitude parameters are vectors, then output is multichannel.
      mask Display: plot([.1 .3 .3001 .4 .4001 .5  .5001 .7],[0 0 1 1 -1 -1 0 0])
  Doublet Generator2 : Subsystem  mask(DoubletGenerator){timeon=10, pulsewidth=40, amplitude=-20}
      mask prompts: timeon "Time Start"; pulsewidth "Pulse Duration"
      mask help:
      | Doublet Generator.
      | Ouputs doublet of specificed amplitude and duration.
      |
      | If start/duration/amplitude parameters are vectors, then output is multichannel.
      mask Display: plot([.1 .3 .3001 .4 .4001 .5  .5001 .7],[0 0 1 1 -1 -1 0 0])
  Gust Generator u_Wg : Subsystem  mask{gust_start=60, gust_duration=15, gust_amplitude=-30}
      mask prompts: gust_start "start time of the gust in sec"; gust_duration "gust duration in sec"; gust_amplitude "maximum gust speed in m/s"
      mask DialogControl ParameterGroupVar Prompt: gust characteristics
  Gust Generator v_Wg : Subsystem  mask{gust_start=20, gust_duration=25, gust_amplitude=-30}
      mask prompts: gust_start "start time of the gust in sec"; gust_duration "gust duration in sec"; gust_amplitude "maximum gust speed in m/s"
      mask DialogControl ParameterGroupVar Prompt: gust characteristics
  Step : Step  Time=10  Before=TrimPoint.States.Psibar  After=deg2rad(10)  SampleTime=0
  Step1 : Step  Time=80  After=deg2rad(170)  SampleTime=0
  Sum : Sum  Inputs=++|
  Sum1 : Sum  Inputs=|++
  Sum2 : Sum  Inputs=++|
  v_Wg : Outport
  u_Wg : Outport  Port=2
  alt_cmd : Outport  Port=3
  Chi_cmd : Outport  Port=4
  beta_cmd : Outport  Port=5
  V_A_cmd : Outport  Port=6
  wires:
  Sum2/1 -> Chi_cmd/1  "Chi_cmd"
  Gust Generator u_Wg/1(wind speed) -> u_Wg/1  "u_Wg"
  Step1/1 -> Sum2/1  "Chi_cmd"
  Constant1/1 -> Sum1/1  "Vabar"
  Step/1 -> Sum2/2  "Chi_cmd"
  Doublet Generator/1(Doublet) -> Sum/1  "alt_cmd"
  Sum/1 -> alt_cmd/1  "alt_cmd"
  Gust Generator v_Wg/1(wind speed) -> v_Wg/1  "v_Wg"
  Doublet Generator2/1(Doublet) -> Sum1/2  "V_A_cmd"
  Constant/1 -> Sum/2  "altbar"
  Doublet Generator1/1(Doublet) -> beta_cmd/1  "beta_cmd"
  Sum1/1 -> V_A_cmd/1  "V_A_cmd"

== system Auxiliary_Models/Test Sequences/Roll Rate Test Sequence ==
  Constant : Constant  Value=TrimPoint.States.Altbar
  Constant1 : Constant  Value=sqrt(TrimPoint.States.ubar^2+TrimPoint.States.vbar^2+TrimPoint.States.wbar^2)
  Constant2 : Constant  Value=0
  Constant3 : Constant  Value=0
  Constant4 : Constant  Value=0
  Sine Wave1 : Sin  Amplitude=ampl_p_cmd  Frequency=omega_p_cmd  SampleTime=0
  v_Wg : Outport
  u_Wg : Outport  Port=2
  alt_cmd : Outport  Port=3
  p_cmd : Outport  Port=4
  beta_cmd : Outport  Port=5
  V_A_cmd : Outport  Port=6
  wires:
  Constant3/1 -> u_Wg/1  "u_Wg"
  Constant1/1 -> V_A_cmd/1  "V_A_cmd"
  Constant2/1 -> beta_cmd/1  "beta_cmd"
  Constant/1 -> alt_cmd/1  "alt_cmd"
  Constant4/1 -> v_Wg/1  "v_Wg"
  Sine Wave1/1 -> p_cmd/1  "p_cmd"

== system Auxiliary_Models/Test Sequences/SAS Test Sequence ==
  Constant : Constant  Value=TrimPoint.States.Altbar
  Constant1 : Constant  Value=sqrt(TrimPoint.States.ubar^2+TrimPoint.States.vbar^2+TrimPoint.States.wbar^2)
  Constant2 : Constant  Value=TrimPoint.States.dabar
  Constant3 : Constant  Value=0
  Gust Generator : Subsystem  mask{gust_start=5, gust_duration=25, gust_amplitude=-30}
      mask prompts: gust_start "start time of the gust in sec"; gust_duration "gust duration in sec"; gust_amplitude "maximum gust speed in m/s"
      mask DialogControl ParameterGroupVar Prompt: gust characteristics
  Step : Step  Time=40  After=deg2rad(5)  SampleTime=0
  v_Wg : Outport
  u_Wg : Outport  Port=2
  alt_cmd : Outport  Port=3
  cmd_da : Outport  Port=4
  cmd_dr : Outport  Port=5
  V_A_cmd : Outport  Port=6
  wires:
  Constant/1 -> alt_cmd/1  "alt_cmd"
  Constant1/1 -> V_A_cmd/1  "V_A_cmd"
  Constant2/1 -> cmd_da/1  "cmd_da"
  Step/1 -> cmd_dr/1  "cmd_dr"
  Gust Generator/1(wind speed) -> v_Wg/1  "v_Wg"
  Constant3/1 -> u_Wg/1  "u_Wg"

== system Auxiliary_Models/Test Sequences/AoS Test Sequence/Gust Generator ==
  1-cos gust : Subsystem  TreatAsAtomicUnit=on
  Clock : Clock
  Compare To Constant : simulink/Logic and Bit Operations/Compare To Constant  relop=>=  const=gust_start  OutDataTypeStr=boolean
  Constant : Constant  Value=0
  Sum : Sum  Inputs=+-|
  Switch : Switch  Criteria=u2 > Threshold  Threshold=gust_start+gust_duration
  time freeze : Subsystem  TreatAsAtomicUnit=on
  wind speed : Outport
  wires:
  time freeze/1(out) -> Sum/2
  Constant/1 -> Switch/1
  Clock/1 -> time freeze/1(in), Compare To Constant/1, Sum/1, Switch/2
  Compare To Constant/1 -> 1-cos gust/Enable, time freeze/Trigger
  Sum/1 -> 1-cos gust/1(in)
  1-cos gust/1(wind) -> Switch/3
  Switch/1 -> wind speed/1

== system Auxiliary_Models/Test Sequences/Bank Angle Test Sequence/Doublet Generator ==
  Add : Sum  Inputs=+++
  DownStep : Step  Time=timeon+pulsewidth  After=-2  SampleTime=0
  Gain : Gain  Gain=amplitude
  UnStep : Step  Time=timeon+2*pulsewidth  SampleTime=0
  UpStep : Step  Time=timeon  SampleTime=0
  Doublet : Outport
  wires:
  UpStep/1 -> Add/1
  DownStep/1 -> Add/2
  UnStep/1 -> Add/3
  Add/1 -> Gain/1
  Gain/1 -> Doublet/1

== system Auxiliary_Models/Test Sequences/Bank Angle Test Sequence/Gust Generator ==
  1-cos gust : Subsystem  TreatAsAtomicUnit=on
  Clock : Clock
  Compare To Constant : simulink/Logic and Bit Operations/Compare To Constant  relop=>=  const=gust_start  OutDataTypeStr=boolean
  Constant : Constant  Value=0
  Sum : Sum  Inputs=+-|
  Switch : Switch  Criteria=u2 > Threshold  Threshold=gust_start+gust_duration
  time freeze : Subsystem  TreatAsAtomicUnit=on
  wind speed : Outport
  wires:
  time freeze/1(out) -> Sum/2
  Constant/1 -> Switch/1
  Clock/1 -> time freeze/1(in), Compare To Constant/1, Sum/1, Switch/2
  Compare To Constant/1 -> 1-cos gust/Enable, time freeze/Trigger
  Sum/1 -> 1-cos gust/1(in)
  1-cos gust/1(wind) -> Switch/3
  Switch/1 -> wind speed/1

== system Auxiliary_Models/Test Sequences/Course Angle Test Sequence/Gust Generator ==
  1-cos gust : Subsystem  TreatAsAtomicUnit=on
  Clock : Clock
  Compare To Constant : simulink/Logic and Bit Operations/Compare To Constant  relop=>=  const=gust_start  OutDataTypeStr=boolean
  Constant : Constant  Value=0
  Sum : Sum  Inputs=+-|
  Switch : Switch  Criteria=u2 > Threshold  Threshold=gust_start+gust_duration
  time freeze : Subsystem  TreatAsAtomicUnit=on
  wind speed : Outport
  wires:
  time freeze/1(out) -> Sum/2
  Constant/1 -> Switch/1
  Clock/1 -> time freeze/1(in), Compare To Constant/1, Sum/1, Switch/2
  Compare To Constant/1 -> 1-cos gust/Enable, time freeze/Trigger
  Sum/1 -> 1-cos gust/1(in)
  1-cos gust/1(wind) -> Switch/3
  Switch/1 -> wind speed/1

== system Auxiliary_Models/Test Sequences/Final Sequence/Doublet Generator ==
  Add : Sum  Inputs=+++
  DownStep : Step  Time=timeon+pulsewidth  After=-2  SampleTime=0
  Gain : Gain  Gain=amplitude
  UnStep : Step  Time=timeon+2*pulsewidth  SampleTime=0
  UpStep : Step  Time=timeon  SampleTime=0
  Doublet : Outport
  wires:
  UpStep/1 -> Add/1
  DownStep/1 -> Add/2
  UnStep/1 -> Add/3
  Add/1 -> Gain/1
  Gain/1 -> Doublet/1

== system Auxiliary_Models/Test Sequences/Final Sequence/Doublet Generator1 ==
  Add : Sum  Inputs=+++
  DownStep : Step  Time=timeon+pulsewidth  After=-2  SampleTime=0
  Gain : Gain  Gain=amplitude
  UnStep : Step  Time=timeon+2*pulsewidth  SampleTime=0
  UpStep : Step  Time=timeon  SampleTime=0
  Doublet : Outport
  wires:
  UpStep/1 -> Add/1
  DownStep/1 -> Add/2
  UnStep/1 -> Add/3
  Add/1 -> Gain/1
  Gain/1 -> Doublet/1

== system Auxiliary_Models/Test Sequences/Final Sequence/Doublet Generator2 ==
  Add : Sum  Inputs=+++
  DownStep : Step  Time=timeon+pulsewidth  After=-2  SampleTime=0
  Gain : Gain  Gain=amplitude
  UnStep : Step  Time=timeon+2*pulsewidth  SampleTime=0
  UpStep : Step  Time=timeon  SampleTime=0
  Doublet : Outport
  wires:
  UpStep/1 -> Add/1
  DownStep/1 -> Add/2
  UnStep/1 -> Add/3
  Add/1 -> Gain/1
  Gain/1 -> Doublet/1

== system Auxiliary_Models/Test Sequences/Final Sequence/Gust Generator u_Wg ==
  1-cos gust : Subsystem  TreatAsAtomicUnit=on
  Clock : Clock
  Compare To Constant : simulink/Logic and Bit Operations/Compare To Constant  relop=>=  const=gust_start  OutDataTypeStr=boolean
  Constant : Constant  Value=0
  Sum : Sum  Inputs=+-|
  Switch : Switch  Criteria=u2 > Threshold  Threshold=gust_start+gust_duration
  time freeze : Subsystem  TreatAsAtomicUnit=on
  wind speed : Outport
  wires:
  time freeze/1(out) -> Sum/2
  Constant/1 -> Switch/1
  Clock/1 -> time freeze/1(in), Compare To Constant/1, Sum/1, Switch/2
  Compare To Constant/1 -> 1-cos gust/Enable, time freeze/Trigger
  Sum/1 -> 1-cos gust/1(in)
  1-cos gust/1(wind) -> Switch/3
  Switch/1 -> wind speed/1

== system Auxiliary_Models/Test Sequences/Final Sequence/Gust Generator v_Wg ==
  1-cos gust : Subsystem  TreatAsAtomicUnit=on
  Clock : Clock
  Compare To Constant : simulink/Logic and Bit Operations/Compare To Constant  relop=>=  const=gust_start  OutDataTypeStr=boolean
  Constant : Constant  Value=0
  Sum : Sum  Inputs=+-|
  Switch : Switch  Criteria=u2 > Threshold  Threshold=gust_start+gust_duration
  time freeze : Subsystem  TreatAsAtomicUnit=on
  wind speed : Outport
  wires:
  time freeze/1(out) -> Sum/2
  Constant/1 -> Switch/1
  Clock/1 -> time freeze/1(in), Compare To Constant/1, Sum/1, Switch/2
  Compare To Constant/1 -> 1-cos gust/Enable, time freeze/Trigger
  Sum/1 -> 1-cos gust/1(in)
  1-cos gust/1(wind) -> Switch/3
  Switch/1 -> wind speed/1

== system Auxiliary_Models/Test Sequences/SAS Test Sequence/Gust Generator ==
  1-cos gust : Subsystem  TreatAsAtomicUnit=on
  Clock : Clock
  Compare To Constant : simulink/Logic and Bit Operations/Compare To Constant  relop=>=  const=gust_start  OutDataTypeStr=boolean
  Constant : Constant  Value=0
  Sum : Sum  Inputs=+-|
  Switch : Switch  Criteria=u2 > Threshold  Threshold=gust_start+gust_duration
  time freeze : Subsystem  TreatAsAtomicUnit=on
  wind speed : Outport
  wires:
  time freeze/1(out) -> Sum/2
  Constant/1 -> Switch/1
  Clock/1 -> time freeze/1(in), Compare To Constant/1, Sum/1, Switch/2
  Compare To Constant/1 -> 1-cos gust/Enable, time freeze/Trigger
  Sum/1 -> 1-cos gust/1(in)
  1-cos gust/1(wind) -> Switch/3
  Switch/1 -> wind speed/1

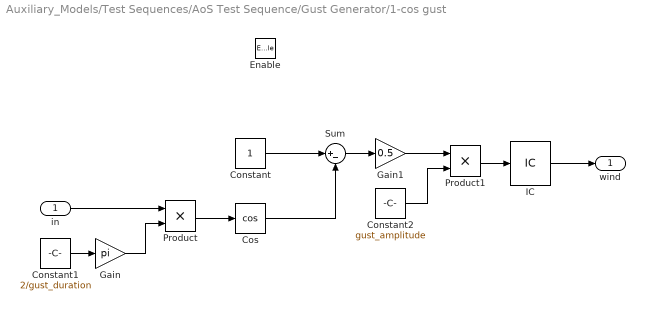
== system Auxiliary_Models/Test Sequences/AoS Test Sequence/Gust Generator/1-cos gust ==
  in : Inport
  Enable : EnablePort  StatesWhenEnabling=reset
  Constant : Constant
  Constant1 : Constant  Value=2/gust_duration
  Constant2 : Constant  Value=gust_amplitude
  Cos : Trigonometry  Operator=cos
  Gain : Gain  Gain=pi
  Gain1 : Gain  Gain=0.5
  IC : InitialCondition  Value=0
  Product : Product
  Product1 : Product
  Sum : Sum  Inputs=|+-
  wind : Outport
  wires:
  IC/1 -> wind/1
  Constant1/1 -> Gain/1
  Product1/1 -> IC/1
  Product/1 -> Cos/1
  Cos/1 -> Sum/2
  Constant/1 -> Sum/1
  Gain/1 -> Product/2
  Gain1/1 -> Product1/1
  Sum/1 -> Gain1/1
  Constant2/1 -> Product1/2
  in/1 -> Product/1

== system Auxiliary_Models/Test Sequences/AoS Test Sequence/Gust Generator/time freeze ==
  in : Inport
  Trigger : TriggerPort  VariantControl=Variant
  out : Outport  InitialOutput=0
  wires:
  in/1 -> out/1

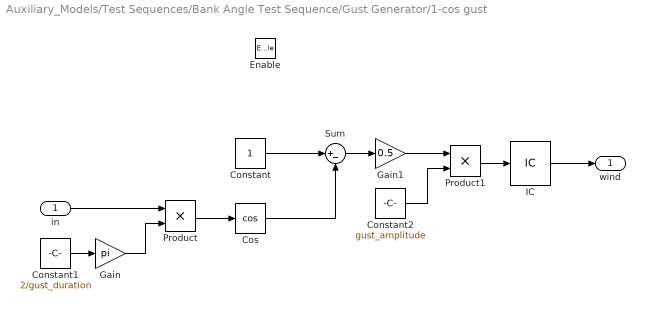
== system Auxiliary_Models/Test Sequences/Bank Angle Test Sequence/Gust Generator/1-cos gust ==
  in : Inport
  Enable : EnablePort  StatesWhenEnabling=reset
  Constant : Constant
  Constant1 : Constant  Value=2/gust_duration
  Constant2 : Constant  Value=gust_amplitude
  Cos : Trigonometry  Operator=cos
  Gain : Gain  Gain=pi
  Gain1 : Gain  Gain=0.5
  IC : InitialCondition  Value=0
  Product : Product
  Product1 : Product
  Sum : Sum  Inputs=|+-
  wind : Outport
  wires:
  IC/1 -> wind/1
  Constant1/1 -> Gain/1
  Product1/1 -> IC/1
  Product/1 -> Cos/1
  Cos/1 -> Sum/2
  Constant/1 -> Sum/1
  Gain/1 -> Product/2
  Gain1/1 -> Product1/1
  Sum/1 -> Gain1/1
  Constant2/1 -> Product1/2
  in/1 -> Product/1

== system Auxiliary_Models/Test Sequences/Bank Angle Test Sequence/Gust Generator/time freeze ==
  in : Inport
  Trigger : TriggerPort  VariantControl=Variant
  out : Outport  InitialOutput=0
  wires:
  in/1 -> out/1

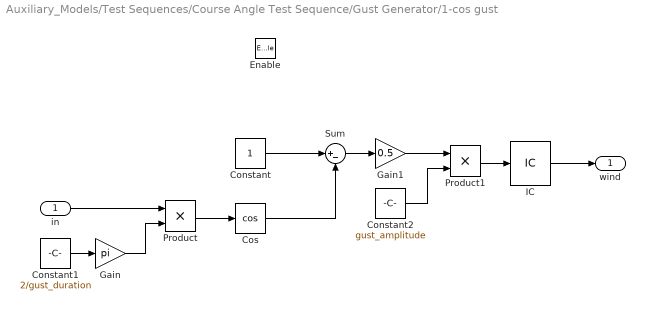
== system Auxiliary_Models/Test Sequences/Course Angle Test Sequence/Gust Generator/1-cos gust ==
  in : Inport
  Enable : EnablePort  StatesWhenEnabling=reset
  Constant : Constant
  Constant1 : Constant  Value=2/gust_duration
  Constant2 : Constant  Value=gust_amplitude
  Cos : Trigonometry  Operator=cos
  Gain : Gain  Gain=pi
  Gain1 : Gain  Gain=0.5
  IC : InitialCondition  Value=0
  Product : Product
  Product1 : Product
  Sum : Sum  Inputs=|+-
  wind : Outport
  wires:
  IC/1 -> wind/1
  Constant1/1 -> Gain/1
  Product1/1 -> IC/1
  Product/1 -> Cos/1
  Cos/1 -> Sum/2
  Constant/1 -> Sum/1
  Gain/1 -> Product/2
  Gain1/1 -> Product1/1
  Sum/1 -> Gain1/1
  Constant2/1 -> Product1/2
  in/1 -> Product/1

== system Auxiliary_Models/Test Sequences/Course Angle Test Sequence/Gust Generator/time freeze ==
  in : Inport
  Trigger : TriggerPort  VariantControl=Variant
  out : Outport  InitialOutput=0
  wires:
  in/1 -> out/1

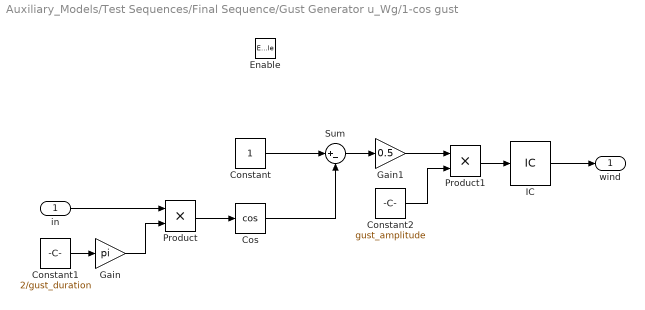
== system Auxiliary_Models/Test Sequences/Final Sequence/Gust Generator u_Wg/1-cos gust ==
  in : Inport
  Enable : EnablePort  StatesWhenEnabling=reset
  Constant : Constant
  Constant1 : Constant  Value=2/gust_duration
  Constant2 : Constant  Value=gust_amplitude
  Cos : Trigonometry  Operator=cos
  Gain : Gain  Gain=pi
  Gain1 : Gain  Gain=0.5
  IC : InitialCondition  Value=0
  Product : Product
  Product1 : Product
  Sum : Sum  Inputs=|+-
  wind : Outport
  wires:
  IC/1 -> wind/1
  Constant1/1 -> Gain/1
  Product1/1 -> IC/1
  Product/1 -> Cos/1
  Cos/1 -> Sum/2
  Constant/1 -> Sum/1
  Gain/1 -> Product/2
  Gain1/1 -> Product1/1
  Sum/1 -> Gain1/1
  Constant2/1 -> Product1/2
  in/1 -> Product/1

== system Auxiliary_Models/Test Sequences/Final Sequence/Gust Generator u_Wg/time freeze ==
  in : Inport
  Trigger : TriggerPort  VariantControl=Variant
  out : Outport  InitialOutput=0
  wires:
  in/1 -> out/1

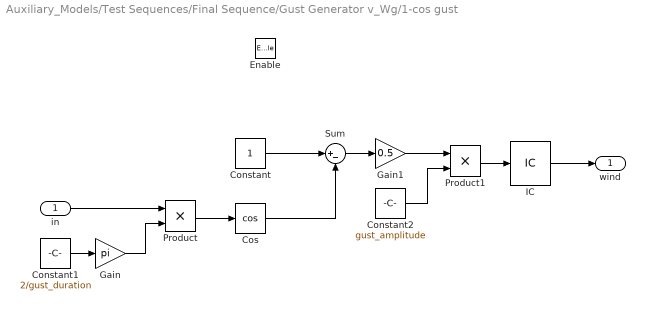
== system Auxiliary_Models/Test Sequences/Final Sequence/Gust Generator v_Wg/1-cos gust ==
  in : Inport
  Enable : EnablePort  StatesWhenEnabling=reset
  Constant : Constant
  Constant1 : Constant  Value=2/gust_duration
  Constant2 : Constant  Value=gust_amplitude
  Cos : Trigonometry  Operator=cos
  Gain : Gain  Gain=pi
  Gain1 : Gain  Gain=0.5
  IC : InitialCondition  Value=0
  Product : Product
  Product1 : Product
  Sum : Sum  Inputs=|+-
  wind : Outport
  wires:
  IC/1 -> wind/1
  Constant1/1 -> Gain/1
  Product1/1 -> IC/1
  Product/1 -> Cos/1
  Cos/1 -> Sum/2
  Constant/1 -> Sum/1
  Gain/1 -> Product/2
  Gain1/1 -> Product1/1
  Sum/1 -> Gain1/1
  Constant2/1 -> Product1/2
  in/1 -> Product/1

== system Auxiliary_Models/Test Sequences/Final Sequence/Gust Generator v_Wg/time freeze ==
  in : Inport
  Trigger : TriggerPort  VariantControl=Variant
  out : Outport  InitialOutput=0
  wires:
  in/1 -> out/1

== system Auxiliary_Models/Test Sequences/SAS Test Sequence/Gust Generator/1-cos gust ==
  in : Inport
  Enable : EnablePort  StatesWhenEnabling=reset
  Constant : Constant
  Constant1 : Constant  Value=2/gust_duration
  Constant2 : Constant  Value=gust_amplitude
  Cos : Trigonometry  Operator=cos
  Gain : Gain  Gain=pi
  Gain1 : Gain  Gain=0.5
  IC : InitialCondition  Value=0
  Product : Product
  Product1 : Product
  Sum : Sum  Inputs=|+-
  wind : Outport
  wires:
  IC/1 -> wind/1
  Constant1/1 -> Gain/1
  Product1/1 -> IC/1
  Product/1 -> Cos/1
  Cos/1 -> Sum/2
  Constant/1 -> Sum/1
  Gain/1 -> Product/2
  Gain1/1 -> Product1/1
  Sum/1 -> Gain1/1
  Constant2/1 -> Product1/2
  in/1 -> Product/1

== system Auxiliary_Models/Test Sequences/SAS Test Sequence/Gust Generator/time freeze ==
  in : Inport
  Trigger : TriggerPort  VariantControl=Variant
  out : Outport  InitialOutput=0
  wires:
  in/1 -> out/1

== matlab function Auxiliary_Models/Choose Shortest Turn ==
  data: e_Chi_in input; e_Chi output
function e_Chi = fcn(e_Chi_in)
%#codegen

if e_Chi_in < -pi
    e_Chi = e_Chi_in + 2*pi;
elseif e_Chi_in > pi
    e_Chi = e_Chi_in - 2*pi;
else
    e_Chi = e_Chi_in;
end

== matlab function Auxiliary_Models/Visualization/wrap Psi to 0-2pi ==
  data: Psi_in input; Psi output
function Psi = fcn(Psi_in)
%#codegen

if Psi_in <0
    Psi = mod(mod(Psi_in+pi,2*pi)+pi,2*pi);
else
    Psi = mod(mod(Psi_in+pi,2*pi)-pi,2*pi);
end
